simulink model "pendule_inv_echant_etu"  (R2021a)
settings: Solver=VariableStepAuto  StartTime=0.0  StopTime=10.0  RelTol=1e-3
values from neighbouring files (symbols this model uses):
  g = 9.81    [simu_pendule_inv_etu.m]
  K = [10 1]    [simu_pendule_inv_etu.m]
  l = 10    [simu_pendule_inv_etu.m]
  t0 = 0    [simu_pendule_inv_etu.m]
  ue = 0    [simu_pendule_inv_etu.m]
  x0 = [pi/20 0]'    [simu_pendule_inv_etu.m]
  xe = [0 0]'    [simu_pendule_inv_etu.m]
undefined symbols (not defined in the file or in its folder): delta_t, DiscIntNeverNeededParam
settings Model: Creator=roussake  LastModifiedBy=roussake

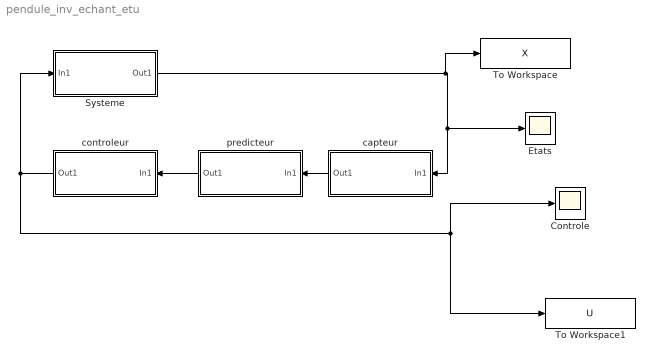
== system pendule_inv_echant_etu ==
  Controle : Scope
  Etats : Scope
  Systeme : Subsystem
  To Workspace : ToWorkspace  VariableName=X  SaveFormat=Timeseries  SampleTime=-1
  To Workspace1 : ToWorkspace  VariableName=U  SaveFormat=Timeseries  SampleTime=-1
  capteur : Subsystem
  controleur : Subsystem
  predicteur : Subsystem
  wires:
  controleur/1(Out1) -> Systeme/1(In1), Controle/1, To Workspace1/1
  Systeme/1(Out1) -> capteur/1(In1), Etats/1, To Workspace/1
  predicteur/1(Out1) -> controleur/1(In1)
  capteur/1(Out1) -> predicteur/1(In1)

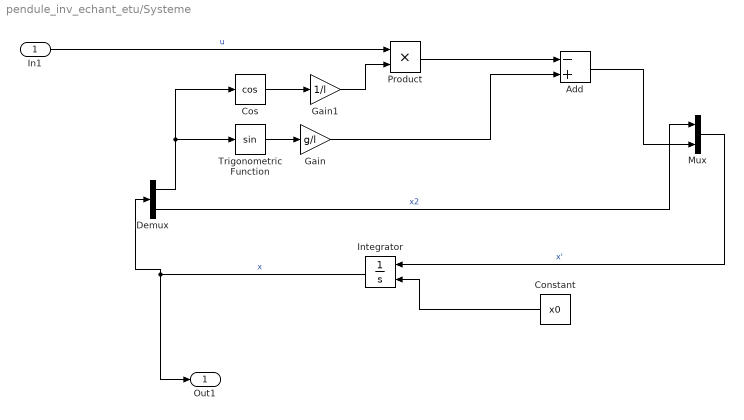
== system pendule_inv_echant_etu/Systeme ==
  In1 : Inport
  Add : Sum  Inputs=-+
  Constant : Constant  Value=x0
  Cos : Trigonometry  Operator=cos
  Demux : Demux  Outputs=2
  Gain : Gain  Gain=g/l
  Gain1 : Gain  Gain=1/l
  Integrator : Integrator  InitialConditionSource=external  InitialCondition=t0
  Mux : Mux  Inputs=2
  Product : Product
  Trigonometric Function : Trigonometry
  Out1 : Outport
  wires:
  Integrator/1 -> Demux/1, Out1/1  "x"
  Demux/2 -> Mux/1  "x2"
  Demux/1 -> Cos/1, Trigonometric Function/1
  Trigonometric Function/1 -> Gain/1
  Cos/1 -> Gain1/1
  In1/1 -> Product/1  "u"
  Gain1/1 -> Product/2
  Product/1 -> Add/1
  Gain/1 -> Add/2
  Add/1 -> Mux/2
  Mux/1 -> Integrator/1  "x'"
  Constant/1 -> Integrator/2

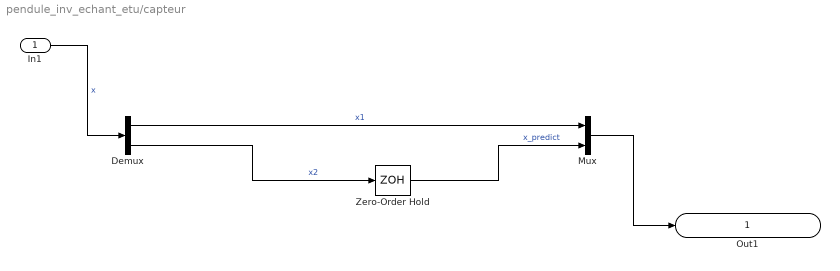
== system pendule_inv_echant_etu/capteur ==
  In1 : Inport
  Demux : Demux  Outputs=2
  Mux : Mux  Inputs=2
  Zero-Order Hold : ZeroOrderHold  SampleTime=delta_t
  Out1 : Outport
  wires:
  In1/1 -> Demux/1  "x"
  Demux/2 -> Zero-Order Hold/1  "x2"
  Zero-Order Hold/1 -> Mux/2  "x_predict"
  Mux/1 -> Out1/1
  Demux/1 -> Mux/1  "x1"

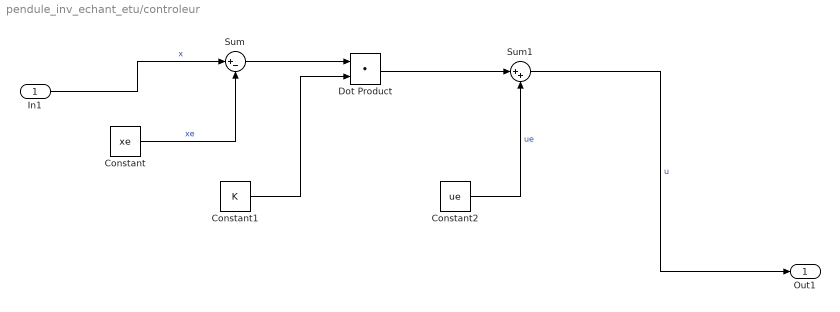
== system pendule_inv_echant_etu/controleur ==
  In1 : Inport
  Constant : Constant  Value=xe
  Constant1 : Constant  Value=K
  Constant2 : Constant  Value=ue
  Dot Product : DotProduct  InputSameDT=on  OutDataTypeStr=Inherit: Inherit via internal rule
  Sum : Sum  Inputs=|+-
  Sum1 : Sum  Inputs=|++
  Out1 : Outport
  wires:
  In1/1 -> Sum/1  "x"
  Constant/1 -> Sum/2  "xe"
  Sum/1 -> Dot Product/1
  Dot Product/1 -> Sum1/1
  Constant2/1 -> Sum1/2  "ue"
  Sum1/1 -> Out1/1  "u"
  Constant1/1 -> Dot Product/2

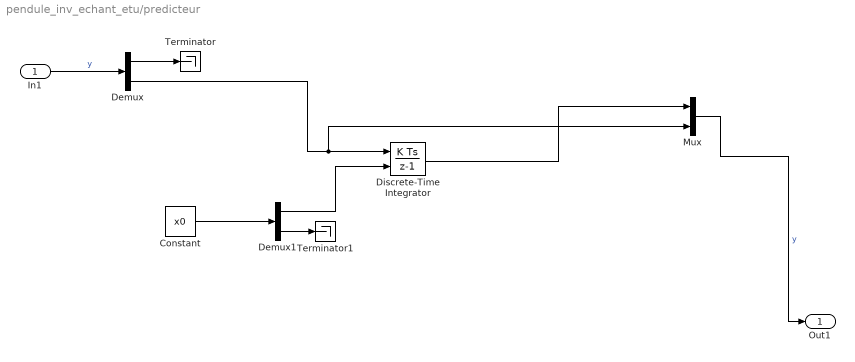
== system pendule_inv_echant_etu/predicteur ==
  In1 : Inport
  Constant : Constant  Value=x0
  Demux : Demux  Outputs=2
  Demux1 : Demux  Outputs=2
  Discrete-Time Integrator : DiscreteIntegrator  InitialConditionSource=external  SampleTime=-1  ICPrevOutput=DiscIntNeverNeededParam  ICPrevScaledInput=DiscIntNeverNeededParam
  Mux : Mux  Inputs=2
  Terminator : Terminator
  Terminator1 : Terminator
  Out1 : Outport
  wires:
  In1/1 -> Demux/1  "y"
  Demux/2 -> Discrete-Time Integrator/1, Mux/2
  Discrete-Time Integrator/1 -> Mux/1
  Constant/1 -> Demux1/1
  Mux/1 -> Out1/1  "y"
  Demux1/1 -> Discrete-Time Integrator/2
  Demux/1 -> Terminator/1
  Demux1/2 -> Terminator1/1
